simulink model "Team_1_Strategy"
settings: Solver=ode45  StartTime=0.0  StopTime=10.0  RelTol=1e-3
settings Model: Creator=smahapat  LastModifiedBy=user
settings SolverCC: ZeroCrossControl=DisableAll
settings DataIOCC: LimitDataPoints=on  SaveFormat=Array  SignalLoggingSaveFormat=ModelDataLogs  ReturnWorkspaceOutputs=off
settings OptimizationCC: InlineParams=on  ExpressionDepthLimit=2147483647  LifeSpan=inf  SimCompilerOptimization=Off
settings DebuggingCC: UnderspecifiedInitializationDetection=Classic  MergeDetectMultiDrivingBlocksExec=none  SolverPrmCheckMsg=warning  FcnCallInpInsideContextMsg=Use local settings  FrameProcessingCompatibilityMsg=warning  StateNameClashWarn=warning  SFUnexpectedBacktrackingDiag=warning  SFNoUnconditionalDefaultTransitionDiag=warning
settings HardwareCC: ProdBitPerPointer=32  ProdLargestAtomicFloat=None  ProdIntDivRoundTo=Undefined  ProdEndianess=Unspecified  ProdWordSize=32  ProdHWDeviceType=32-bit Generic
settings ModelReferenceCC: PropagateSignalLabelsOutOfModel=off
settings SFSimCC: SimUseLocalCustomCode=off  SimParseCustomCode=off
settings RTWCC: RTWUseLocalCustomCode=off  RTWCompilerOptimization=Off
settings CodeAppCC: CustomSymbolStrType=$N$R$M
settings GRTTargetCC: CodeReplacementLibrary=ANSI_C  GeneratePreprocessorConditionals=Disable all  CombineOutputUpdateFcns=off  CPPClassGenCompliant=off  GRTInterface=on

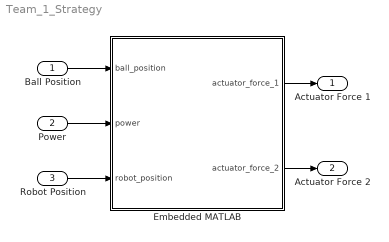
== system Team_1_Strategy ==
  Ball Position : Inport  PortDimensions=[2 1]
  Power : Inport  Port=2  PortDimensions=[4 1]  BusOutputAsStruct=on
  Robot Position : Inport  Port=3  PortDimensions=[8 1]  BusOutputAsStruct=on
  Embedded MATLAB : MATLAB Function  TreatAsAtomicUnit=on
  " Actuator Force 1" : Outport
  Actuator Force 2 : Outport  Port=2
  wires:
  Ball Position/1 -> Embedded MATLAB/1(ball_position)
  Robot Position/1 -> Embedded MATLAB/3(robot_position)
  Embedded MATLAB/1(actuator_force_1) -> " Actuator Force 1"/1
  Embedded MATLAB/2(actuator_force_2) -> Actuator Force 2/1
  Power/1 -> Embedded MATLAB/2(power)

== matlab function Team_1_Strategy/Embedded MATLAB ==
  data: ball_position input; power input; actuator_force_1 output; robot_position input; actuator_force_2 output
function [actuator_force_1, actuator_force_2] = fcn(ball_position, power,  robot_position)
%#eml

d1=(robot_position(1:2,1)-ball_position);
d2=(robot_position(3:4,1)-ball_position);
if dot(d1,d1)>5
   actuator_force_1=-22*d1;
else
   r1=(ball_position- [200;50]);
   actuator_force_1=-11*r1;
end
if dot(d2,d2)>5
   actuator_force_2=-25*d2;
else
   r2=(ball_position-[200;50]);
   actuator_force_2=-15*r2;
end
